simulink model "invertedPendolum"  (R2019a)
settings: Solver=VariableStepAuto  StartTime=0.0  StopTime=30  FixedStep=0.0001  RelTol=1e-3
InitFcn:
  | simulationVar
undefined symbols (not defined in the file): kMot
libraries: simulink x2
settings Model: Creator=alfyhack  LastModifiedBy=alfyhack
settings SolverCC: AlgebraicLoopSolver=LineSearch
settings DebuggingCC: UnderSpecifiedDimensionMsg=warning

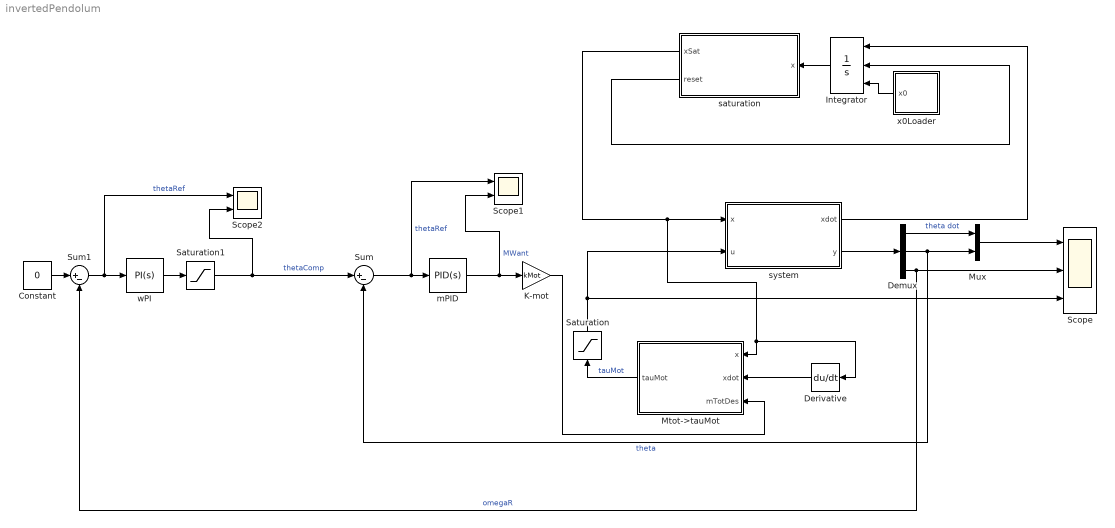
== system invertedPendolum ==
  Constant : Constant  Value=0
  Demux : Demux  Outputs=3
  Derivative : Derivative  CoefficientInTFapproximation=100
  Integrator : Integrator  ExternalReset=rising  InitialConditionSource=external  InitialCondition=[0,0.1,0]
  K-mot : Gain  Gain=kMot
  Mtot->tauMot : MATLAB Function  TreatAsAtomicUnit=on
  Mux : Mux  Inputs=2
  Saturation : Saturate  UpperLimit=0.9*10^9  LowerLimit=-0.9*10^9
  Saturation1 : Saturate  UpperLimit=10  LowerLimit=-10
  Scope : Scope  NumInputPorts=3
  Scope1 : Scope  NumInputPorts=2
  Scope2 : Scope  NumInputPorts=2
  Sum : Sum  Inputs=|+-
  Sum1 : Sum  Inputs=|+-
  mPID : simulink/Continuous/PID Controller  Controller=PID  Form=Parallel  TimeDomain=Continuous-time  SampleTime=-1  IntegratorMethod=Forward Euler  FilterMethod=Forward Euler  ControllerParametersSource=internal  P=-500000000  I=-400000  D=-20000000  UseFilter=on  N=2000  TunerSelectOption=Transfer Function Based (PID Tuner App)  InitialConditionSource=internal  InitialConditionForIntegrator=0  InitialConditionForFilter=0  DifferentiatorICPrevScaledInput=0  ExternalReset=none  TrackingMode=off  Kt=1  LimitOutput=off  UpperSaturationLimit=1000  LowerSaturationLimit=1000  LinearizeAsGain=off  AntiWindupMode=none  Kb=1  POutMin=[]  POutMax=[]  IOutMin=[]  IOutMax=[]  DOutMin=[]  DOutMax=[]  NOutMin=[]  NOutMax=[]  SumOutMin=[]  SumOutMax=[]  SaturationOutMin=[]  SaturationOutMax=[]  PParamMin=[]  PParamMax=[]  IParamMin=[]  IParamMax=[]  DParamMin=[]  DParamMax=[]  NParamMin=[]  NParamMax=[]  KbParamMin=[]  KbParamMax=[]  KtParamMin=[]  KtParamMax=[]  KbOutMin=[]  KbOutMax=[]  KtOutMin=[]  KtOutMax=[]  IntegratorOutMin=[]  IntegratorOutMax=[]  FilterOutMin=[]  FilterOutMax=[]  SumI1OutMin=[]  SumI1OutMax=[]  SumI2OutMin=[]  SumI2OutMax=[]  SumI3OutMin=[]  SumI3OutMax=[]  SumI4OutMin=[]  SumI4OutMax=[]  SumDOutMin=[]  SumDOutMax=[]  DifferentiatorOutMin=[]  DifferentiatorOutMax=[]  FilterDiffOutCoefMin=[]  FilterDiffOutCoefMax=[]  ReciprocalOutMin=[]  ReciprocalOutMax=[]  SumDenOutMin=[]  SumDenOutMax=[]  SumNumOutMin=[]  SumNumOutMax=[]  DivideOutMin=[]  DivideOutMax=[]  IntegratorContinuousStateAttributes=''  IntegratorStateMustResolveToSignalObject=off  IntegratorRTWStateStorageClass=Auto  FilterContinuousStateAttributes=''  FilterStateMustResolveToSignalObject=off  FilterRTWStateStorageClass=Auto  ParallelPVariant=InternalParameters  IdealPVariant=Disabled  IVariant=InternalParameters  DVariant=InternalParameters  IntegratorVariant=Continuous  SatVariant=Disabled  AWVariant=Passthrough  PCopyVariant=Disabled  TRVariant=Disabled  FdbkBlocksVariant=Forward  IdealPFdbkVariant=Disabled  SatFdbkVariant=Disabled  DerivativeFilterVariant=ContFilter  NVariant=InternalParameters  NCopyVariant=Disabled  FilterICVariant=InternalICsFilter  IntegratorICVariant=InternalICs  ExternalResetVariant=Disabled  TRSumVariant=Passthrough  SumFdbkVariant=Disabled  SumVariant=Sum_PID
  saturation : MATLAB Function  TreatAsAtomicUnit=on
  system : MATLAB Function  TreatAsAtomicUnit=on
  wPI : simulink/Continuous/PID Controller  Controller=PI  Form=Parallel  TimeDomain=Continuous-time  SampleTime=-1  IntegratorMethod=Forward Euler  FilterMethod=Forward Euler  ControllerParametersSource=internal  P=0.00405445865250515  I=3.17860947444756e-05  D=1  UseFilter=on  N=2000  TunerSelectOption=Transfer Function Based (PID Tuner App)  InitialConditionSource=internal  InitialConditionForIntegrator=0  InitialConditionForFilter=0  DifferentiatorICPrevScaledInput=0  ExternalReset=none  TrackingMode=off  Kt=1  LimitOutput=off  UpperSaturationLimit=10  LowerSaturationLimit=-10  LinearizeAsGain=off  AntiWindupMode=none  Kb=1  POutMin=[]  POutMax=[]  IOutMin=[]  IOutMax=[]  DOutMin=[]  DOutMax=[]  NOutMin=[]  NOutMax=[]  SumOutMin=[]  SumOutMax=[]  SaturationOutMin=[]  SaturationOutMax=[]  PParamMin=[]  PParamMax=[]  IParamMin=[]  IParamMax=[]  DParamMin=[]  DParamMax=[]  NParamMin=[]  NParamMax=[]  KbParamMin=[]  KbParamMax=[]  KtParamMin=[]  KtParamMax=[]  KbOutMin=[]  KbOutMax=[]  KtOutMin=[]  KtOutMax=[]  IntegratorOutMin=[]  IntegratorOutMax=[]  FilterOutMin=[]  FilterOutMax=[]  SumI1OutMin=[]  SumI1OutMax=[]  SumI2OutMin=[]  SumI2OutMax=[]  SumI3OutMin=[]  SumI3OutMax=[]  SumI4OutMin=[]  SumI4OutMax=[]  SumDOutMin=[]  SumDOutMax=[]  DifferentiatorOutMin=[]  DifferentiatorOutMax=[]  FilterDiffOutCoefMin=[]  FilterDiffOutCoefMax=[]  ReciprocalOutMin=[]  ReciprocalOutMax=[]  SumDenOutMin=[]  SumDenOutMax=[]  SumNumOutMin=[]  SumNumOutMax=[]  DivideOutMin=[]  DivideOutMax=[]  IntegratorContinuousStateAttributes=''  IntegratorStateMustResolveToSignalObject=off  IntegratorRTWStateStorageClass=Auto  FilterContinuousStateAttributes=''  FilterStateMustResolveToSignalObject=off  FilterRTWStateStorageClass=Auto  ParallelPVariant=InternalParameters  IdealPVariant=Disabled  IVariant=InternalParameters  DVariant=Disabled  IntegratorVariant=Continuous  SatVariant=Disabled  AWVariant=Passthrough  PCopyVariant=Disabled  TRVariant=Disabled  FdbkBlocksVariant=Forward  IdealPFdbkVariant=Disabled  SatFdbkVariant=Disabled  DerivativeFilterVariant=Disabled  NVariant=Disabled  NCopyVariant=Disabled_SignalSpec  FilterICVariant=Disabled  IntegratorICVariant=InternalICs  ExternalResetVariant=Disabled  TRSumVariant=Passthrough  SumFdbkVariant=Disabled  SumVariant=Sum_PI
  x0Loader : MATLAB Function  TreatAsAtomicUnit=on
  wires:
  system/1(xdot) -> Integrator/1
  system/2(y) -> Demux/1
  Demux/2 -> Mux/2, Sum/2  "theta"
  Demux/1 -> Mux/1  "theta dot"
  Mux/1 -> Scope/1
  Demux/3 -> Sum1/2, Scope/2  "omegaR"
  Mtot->tauMot/1(tauMot) -> Saturation/1  "tauMot"
  Integrator/1 -> saturation/1(x)
  saturation/2(reset) -> Integrator/2
  saturation/1(xSat) -> Mtot->tauMot/1(x), Derivative/1, system/1(x)
  x0Loader/1(x0) -> Integrator/3
  mPID/1 -> K-mot/1, Scope1/2  "MWant"
  Sum/1 -> Scope1/1, mPID/1  "thetaRef"
  wPI/1 -> Saturation1/1
  Derivative/1 -> Mtot->tauMot/2(xdot)
  Saturation/1 -> Scope/3, system/2(u)
  K-mot/1 -> Mtot->tauMot/3(mTotDes)
  Saturation1/1 -> Sum/1, Scope2/2  "thetaComp"
  Constant/1 -> Sum1/1
  Sum1/1 -> Scope2/1, wPI/1  "thetaRef"

== matlab function invertedPendolum/system ==
  data: x input; xdot output; u input; y output
function [xdot,y] = pendoloNotLinSys(x,u)
%PENDOLONOTLINSYS Summary of this function goes here
% x1:= theta dot    [rad/s]
% x2:= theta        [rad]
% x3:= omegaR       [rad/s]
% u:= Coppia motore [g/s^2 * mm]

coder.extrinsic('evalin', 'assignin')
g = 0;                  % Needed in order to set variable class correctly
g = evalin('base','g'); % Read value from workspace

mCm = 0;                  % Needed in order to set variable class correctly
mCm = evalin('base','mCm'); % Read value from workspace

Lcm = 0;                  % Needed in order to set variable class correctly
Lcm = evalin('base','Lcm'); % Read value from workspace

It = 0;                  % Needed in order to set variable class correctly
It = evalin('base','It'); % Read value from workspace

Ia = 0;                  % Needed in order to set variable class correctly
Ia = evalin('base','Ia'); % Read value from workspace

thetaMax = 0;                  % Needed in order to set variable class correctly
thetaMax = evalin('base','thetaMax'); % Read value from workspace

% Calcoli notevoli:
Mg = (mCm*g*Lcm/It)*sin(x(2));

xdot=zeros(3,1);
% x1dot:= theta 2 dot
xdot(1) = Mg - (1/It)*u;
% if((abs(x(2))>=thetaMax))    %reazione vincolare
%     xdot(1) = xdot(1) + Mg;
% end
xdot(1) = xdot(1) - 1*x(1); %attrito viscoso
% if(abs(xdot(1))<=0.1)
%     xdot(1)=0;              % errore numerico
% end

% x2dot:= theta dot
xdot(2) = x(1);
% x3dot:= omegaR dot
xdot(3) = -xdot(1) + (1/Ia)*u;


%per ora supponiamo di poter osservare tutto il sistema
y=x;

end

== matlab function invertedPendolum/saturation ==
  data: x input; xSat output; reset output
function [xSat,reset]  = phisicReaction(x)
%PHISICREACTION Summary of this function goes here
% Funzione che letto lo stato, in caso di urto con la base cambia
% in maniera realistica lo stato introducendo una saturazione.
% x1:= theta dot    [rad/s]
% x2:= theta        [rad]
% x3:= omegaR       [rad/s]

coder.extrinsic('evalin', 'assignin')
thetaMax = 0;                  % Needed in order to set variable class correctly
thetaMax = evalin('base','thetaMax'); % Read value from workspace

xSat=x;
if((abs(x(2))>thetaMax)&&(sign(x(1))==sign(x(2))))
    
    xSat(1)=-x(1)*0.5;      % dissopazione di energia
%     if(abs(xSat(1))<=0.1)
%         xSat(1)=0;              % errore numerico
%     end
    
    xSat(2)=sign(x(2))*thetaMax; %riposizionamento
    
    %to reset integrator state
    assignin('base','x0',xSat); % Assign value back to workspace
    reset=1;
else
    reset=0;
end

end

== matlab function invertedPendolum/x0Loader ==
  data: x0 output
function x0 = loadX0()
coder.extrinsic('evalin', 'assignin')
x0 = zeros(3,1);          % Needed in order to set variable class correctly
x0 = evalin('base','x0'); % Read value from workspace

== matlab function invertedPendolum/Mtot->tauMot ==
  data: x input; tauMot output; xdot input; mTotDes input
function tauMot = mTot2mMot(x,xdot, mTotDes)
% x1:= theta dot    [rad/s]
% x2:= theta        [rad]
% x3:= omegaR       [rad/s]
% tauMot:= Coppia motore [g/s^2 * mm]

% x1dot:= theta 2 dot   [rad/s^21]
% x2dot:= theta dot     [rad/s]
% x3dot:= omegaR dot    [rad/s^2]

coder.extrinsic('evalin', 'assignin')
g = 0;                  % Needed in order to set variable class correctly
g = evalin('base','g'); % Read value from workspace

mCm = 0;                  % Needed in order to set variable class correctly
mCm = evalin('base','mCm'); % Read value from workspace

Lcm = 0;                  % Needed in order to set variable class correctly
Lcm = evalin('base','Lcm'); % Read value from workspace

It = 0;                  % Needed in order to set variable class correctly
It = evalin('base','It'); % Read value from workspace

% Calcoli notevoli:
Mg = (mCm*g*Lcm/It)*sin(x(2));
% tauMot = Mdes- Mattuale
tauMot = mTotDes-(Mg-It*xdot(1));

end
